simulink model "PDPWM_Three_Phase_Three_Level_Clamped_Inverter"  (R2022a)
settings: Solver=FixedStepAuto  StartTime=0.0  StopTime=0.3  FixedStep=1e-5  RelTol=1e-3
libraries: spsIGBTDiodeLib x12, spsDiodeLib x6, simulink x6, spsSeriesRLCBranchLib x5, spsGroundLib x2, spsDCVoltageSourceLib x1, spsThreePhaseVIMeasurementLib x1, spspowerguiLib x1
settings Model: Creator=nikos  LastModifiedBy=nikos

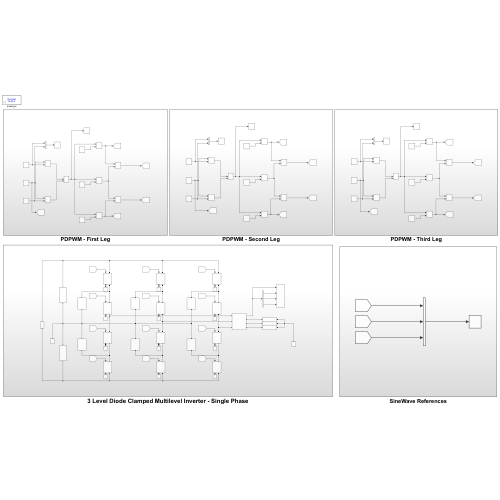
[thumbnail: Simulink's stored preview of the top-level diagram]
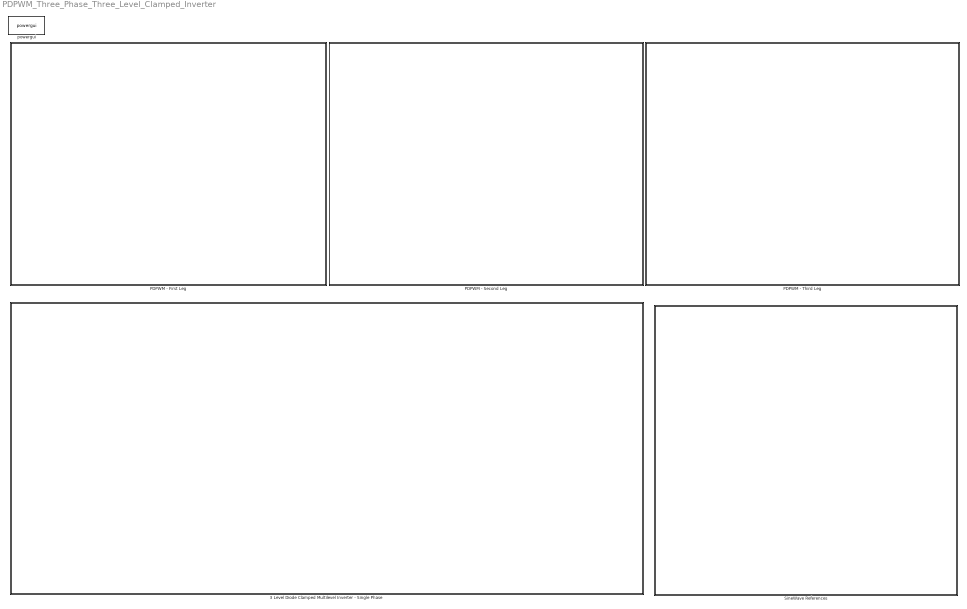
== system PDPWM_Three_Phase_Three_Level_Clamped_Inverter ==
  3 Level Diode Clamped Multilevel Inverter - Single Phase : Subsystem
  PDPWM - First Leg : Subsystem
  PDPWM - Second Leg : Subsystem
  PDPWM - Third Leg : Subsystem
  SineWave References : Subsystem
  powergui : spspowerguiLib/powergui  Priority=1  SimulationMode=Discrete  SampleTime=1e-5  frequency=60  Iterations=50  frequencyindice=0  Pbase=100e6  ErrMax=1e-4  UnitsV=kV  UnitsW=MW  buscounter=0  FunctionMessages=off  echomessages=off  EnableUseOfTLC=off  CurrentSourceSwitches=off  DisableSnubberDevices=off  DisableRonSwitches=off  DisableVfSwitches=off  DisplayEquations=off  AutomaticDiscreteSolvers=off  SolverType=Tustin/Backward Euler (TBE)  Interpol=off  ExternalGateDelay=off  methode=off  Ts=100  x0status=blocks  SPID=on  SwTol=0  HookPort=off  NonlinearTolerance=1e-4  nMaxIteration=100  ContinueOnMaxIteration=off  RestoreLinks=warning  ResistiveCurrentMeasurement=off  Frange=[0:2:500]  Ylog=off  Xlog=on  ShowGrid=off  save=off  variable=ZData  structure=0  ZoomFFT=off  StartTime=0.0  cycles=1  DisplayStyle=1  fundamental=60  FreqAxis=off  MaxFrequency=1000  frequencyindicesteady=1  RmsSteady=1  display=off

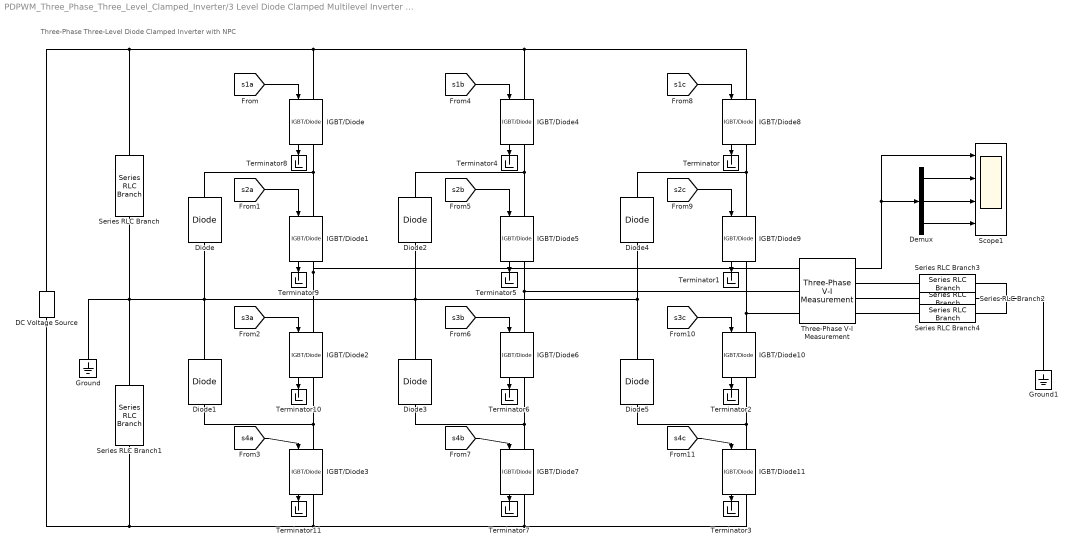
== system PDPWM_Three_Phase_Three_Level_Clamped_Inverter/3 Level Diode Clamped Multilevel Inverter - Single Phase ==
  note: Three-Phase Three-Level Diode Clamped Inverter with NPC
  DC Voltage Source : spsDCVoltageSourceLib/DC Voltage Source  Amplitude=100  Measurements=None
  Demux : Demux  Outputs=3
  Diode{,1..5} (6 alike) : spsDiodeLib/Diode  Ron=0.001  Lon=0  Vf=0.8  IC=0  UseSnubber=0  Rs=500  Cs=250e-9  Measurements=off
  Ground : spsGroundLib/Ground  LConnTagsString=a
  Ground1 : spsGroundLib/Ground  LConnTagsString=a
  IGBT/Diode{,1..11} (12 alike) : spsIGBTDiodeLib/IGBT//Diode  Ron=1e-3  Rs=1e5  Cs=inf  Measurements=on
  Scope1 : Scope  NumInputPorts=4
  Series RLC Branch : spsSeriesRLCBranchLib/Series RLC Branch  LConnTagsString=__new0  RConnTagsString=__new0  BranchType=RC  Resistance=0.01  Inductance=1e-3  SetiL0=off  InitialCurrent=0  Capacitance=4.7e-3  Setx0=off  InitialVoltage=0  Measurements=None
  Series RLC Branch1 : spsSeriesRLCBranchLib/Series RLC Branch  LConnTagsString=__new0  RConnTagsString=__new0  BranchType=RC  Resistance=0.01  Inductance=1e-3  SetiL0=off  InitialCurrent=0  Capacitance=4.7e-3  Setx0=off  InitialVoltage=0  Measurements=None
  Series RLC Branch2 : spsSeriesRLCBranchLib/Series RLC Branch  LConnTagsString=__new0  RConnTagsString=__new0  BranchType=R  Resistance=100  Inductance=1e-3  SetiL0=off  InitialCurrent=0  Capacitance=1e-6  Setx0=off  InitialVoltage=0  Measurements=None
  Series RLC Branch3 : spsSeriesRLCBranchLib/Series RLC Branch  LConnTagsString=__new0  RConnTagsString=__new0  BranchType=R  Resistance=100  Inductance=1e-3  SetiL0=off  InitialCurrent=0  Capacitance=1e-6  Setx0=off  InitialVoltage=0  Measurements=None
  Series RLC Branch4 : spsSeriesRLCBranchLib/Series RLC Branch  LConnTagsString=__new0  RConnTagsString=__new0  BranchType=R  Resistance=100  Inductance=1e-3  SetiL0=off  InitialCurrent=0  Capacitance=1e-6  Setx0=off  InitialVoltage=0  Measurements=None
  Terminator{,1..11} (12 alike) : Terminator
  Three-Phase V-I Measurement : spsThreePhaseVIMeasurementLib/Three-Phase V-I Measurement  VoltageMeasurement=phase-to-ground  SetLabelV=off  LabelV=Vabc  Vpu=off  VpuLL=off  CurrentMeasurement=no  SetLabelI=off  LabelI=Iabc  Ipu=off  Pbase=100e6  Vbase=500e3  OutputType=Complex  PhasorSimulation=off  PSBequivalent=0
  wires:
  [s4b] -> IGBT/Diode7/1
  [s2c] -> IGBT/Diode9/1
  Three-Phase V-I Measurement/1 -> Demux/1, Scope1/1
  Demux/3 -> Scope1/4
  [s3a] -> IGBT/Diode2/1
  [s3b] -> IGBT/Diode6/1
  [s2b] -> IGBT/Diode5/1
  [s1b] -> IGBT/Diode4/1
  [s4c] -> IGBT/Diode11/1
  [s2a] -> IGBT/Diode1/1
  [s1c] -> IGBT/Diode8/1
  [s1a] -> IGBT/Diode/1
  [s4a] -> IGBT/Diode3/1
  [s3c] -> IGBT/Diode10/1
  Demux/1 -> Scope1/2
  Demux/2 -> Scope1/3
  IGBT/Diode8/1 -> Terminator/1
  IGBT/Diode9/1 -> Terminator1/1
  IGBT/Diode10/1 -> Terminator2/1
  IGBT/Diode4/1 -> Terminator4/1
  IGBT/Diode5/1 -> Terminator5/1
  IGBT/Diode6/1 -> Terminator6/1
  IGBT/Diode7/1 -> Terminator7/1
  IGBT/Diode/1 -> Terminator8/1
  IGBT/Diode1/1 -> Terminator9/1
  IGBT/Diode2/1 -> Terminator10/1
  IGBT/Diode3/1 -> Terminator11/1
  IGBT/Diode11/1 -> Terminator3/1
  connections:
  IGBT/Diode7/LConn1 -- IGBT/Diode6/RConn1 -- Diode3/LConn1
  IGBT/Diode/RConn1 -- Diode/RConn1 -- IGBT/Diode1/LConn1
  Series RLC Branch1/RConn1 -- DC Voltage Source/LConn1 -- IGBT/Diode3/RConn1 -- IGBT/Diode7/RConn1 -- IGBT/Diode11/RConn1
  IGBT/Diode9/RConn1 -- Three-Phase V-I Measurement/LConn3 -- IGBT/Diode10/LConn1
  IGBT/Diode2/RConn1 -- Diode1/LConn1 -- IGBT/Diode3/LConn1
  IGBT/Diode5/LConn1 -- IGBT/Diode4/RConn1 -- Diode2/RConn1
  Series RLC Branch/RConn1 -- Ground/LConn1 -- Diode4/LConn1 -- Diode5/RConn1 -- Diode2/LConn1 -- Diode3/RConn1 -- Diode/LConn1 -- Diode1/RConn1 -- Series RLC Branch1/LConn1
  IGBT/Diode1/RConn1 -- IGBT/Diode2/LConn1 -- Three-Phase V-I Measurement/LConn1
  Series RLC Branch/LConn1 -- DC Voltage Source/RConn1 -- IGBT/Diode/LConn1 -- IGBT/Diode4/LConn1 -- IGBT/Diode8/LConn1
  IGBT/Diode5/RConn1 -- Three-Phase V-I Measurement/LConn2 -- IGBT/Diode6/LConn1
  IGBT/Diode10/RConn1 -- IGBT/Diode11/LConn1 -- Diode5/LConn1
  IGBT/Diode8/RConn1 -- IGBT/Diode9/LConn1 -- Diode4/RConn1
  Ground1/LConn1 -- Series RLC Branch4/LConn1 -- Series RLC Branch3/LConn1 -- Series RLC Branch2/LConn1
  Three-Phase V-I Measurement/RConn1 -- Series RLC Branch3/RConn1
  Three-Phase V-I Measurement/RConn3 -- Series RLC Branch4/RConn1
  Three-Phase V-I Measurement/RConn2 -- Series RLC Branch2/RConn1

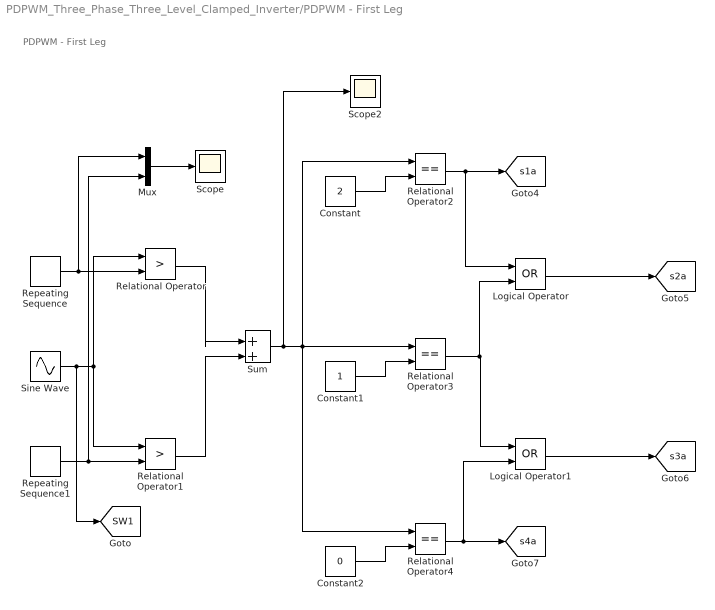
== system PDPWM_Three_Phase_Three_Level_Clamped_Inverter/PDPWM - First Leg ==
  note: PDPWM - First Leg
  Constant : Constant  Value=2
  Constant1 : Constant
  Constant2 : Constant  Value=0
  Logical Operator : Logic  Operator=OR  AllPortsSameDT=off  OutDataTypeStr=boolean
  Logical Operator1 : Logic  Operator=OR  AllPortsSameDT=off  OutDataTypeStr=boolean
  Mux : Mux  Inputs=2
  Relational Operator : RelationalOperator  Operator=>  OutDataTypeStr=boolean  RndMeth=Simplest  InputSameDT=off
  Relational Operator1 : RelationalOperator  Operator=>  OutDataTypeStr=boolean  RndMeth=Simplest  InputSameDT=off
  Relational Operator2 : RelationalOperator  Operator===  OutDataTypeStr=boolean  RndMeth=Simplest  InputSameDT=off
  Relational Operator3 : RelationalOperator  Operator===  OutDataTypeStr=boolean  RndMeth=Simplest  InputSameDT=off
  Relational Operator4 : RelationalOperator  Operator===  OutDataTypeStr=boolean  RndMeth=Simplest  InputSameDT=off
  Repeating Sequence : simulink/Sources/Repeating Sequence  rep_seq_t=[0 1 2]*[1/1000]  rep_seq_y=[0 1 0]
  Repeating Sequence1 : simulink/Sources/Repeating Sequence  rep_seq_t=[0 1 2]*[1/1000]  rep_seq_y=[-1 0 -1]
  Scope : Scope
  Scope2 : Scope
  Sine Wave : Sin  Frequency=2*pi*50  SampleTime=0
  Sum : Sum  Inputs=|++
  tag scope: SW1=global, s1a=global, s2a=global, s3a=global, s4a=global
  wires:
  Relational Operator3/1 -> Logical Operator/2, Logical Operator1/1
  Constant/1 -> Relational Operator2/2
  Repeating Sequence/1 -> Mux/1, Relational Operator/2
  Repeating Sequence1/1 -> Relational Operator1/2, Mux/2
  Relational Operator4/1 -> [s4a], Logical Operator1/2
  Relational Operator/1 -> Sum/1
  Relational Operator1/1 -> Sum/2
  Sine Wave/1 -> [SW1], Relational Operator1/1, Relational Operator/1
  Relational Operator2/1 -> [s1a], Logical Operator/1
  Mux/1 -> Scope/1
  Sum/1 -> Scope2/1, Relational Operator4/1, Relational Operator2/1, Relational Operator3/1
  Logical Operator/1 -> [s2a]
  Constant2/1 -> Relational Operator4/2
  Constant1/1 -> Relational Operator3/2
  Logical Operator1/1 -> [s3a]

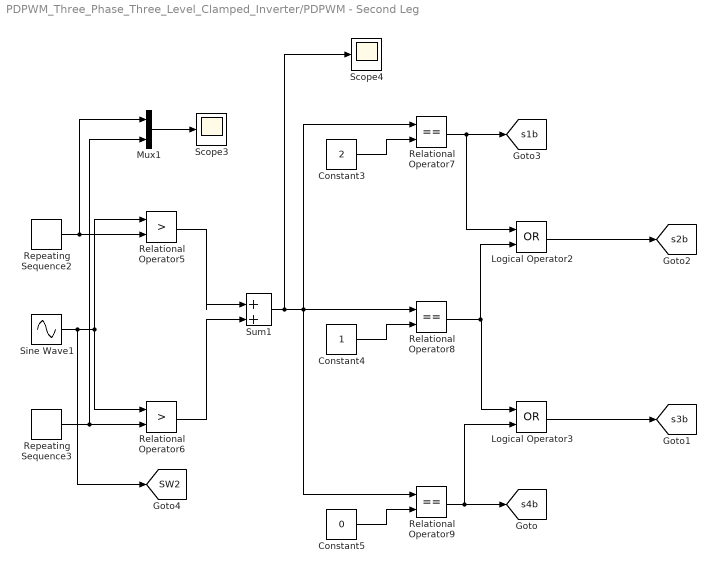
== system PDPWM_Three_Phase_Three_Level_Clamped_Inverter/PDPWM - Second Leg ==
  Constant3 : Constant  Value=2
  Constant4 : Constant
  Constant5 : Constant  Value=0
  Logical Operator2 : Logic  Operator=OR  AllPortsSameDT=off  OutDataTypeStr=boolean
  Logical Operator3 : Logic  Operator=OR  AllPortsSameDT=off  OutDataTypeStr=boolean
  Mux1 : Mux  Inputs=2
  Relational Operator5 : RelationalOperator  Operator=>  OutDataTypeStr=boolean  RndMeth=Simplest  InputSameDT=off
  Relational Operator6 : RelationalOperator  Operator=>  OutDataTypeStr=boolean  RndMeth=Simplest  InputSameDT=off
  Relational Operator7 : RelationalOperator  Operator===  OutDataTypeStr=boolean  RndMeth=Simplest  InputSameDT=off
  Relational Operator8 : RelationalOperator  Operator===  OutDataTypeStr=boolean  RndMeth=Simplest  InputSameDT=off
  Relational Operator9 : RelationalOperator  Operator===  OutDataTypeStr=boolean  RndMeth=Simplest  InputSameDT=off
  Repeating Sequence2 : simulink/Sources/Repeating Sequence  rep_seq_t=[0 1 2]*[1/1000]  rep_seq_y=[0 1 0]
  Repeating Sequence3 : simulink/Sources/Repeating Sequence  rep_seq_t=[0 1 2]*[1/1000]  rep_seq_y=[-1 0 -1]
  Scope3 : Scope
  Scope4 : Scope
  Sine Wave1 : Sin  Frequency=2*pi*50  Phase=4*pi/3  SampleTime=0
  Sum1 : Sum  Inputs=|++
  tag scope: SW2=global, s1b=global, s2b=global, s3b=global, s4b=global
  wires:
  Sum1/1 -> Relational Operator8/1, Relational Operator7/1, Relational Operator9/1, Scope4/1
  Relational Operator6/1 -> Sum1/2
  Relational Operator7/1 -> [s1b], Logical Operator2/1
  Logical Operator3/1 -> [s3b]
  Relational Operator5/1 -> Sum1/1
  Sine Wave1/1 -> [SW2], Relational Operator5/1, Relational Operator6/1
  Logical Operator2/1 -> [s2b]
  Relational Operator9/1 -> [s4b], Logical Operator3/2
  Relational Operator8/1 -> Logical Operator3/1, Logical Operator2/2
  Repeating Sequence3/1 -> Mux1/2, Relational Operator6/2
  Mux1/1 -> Scope3/1
  Constant3/1 -> Relational Operator7/2
  Constant4/1 -> Relational Operator8/2
  Constant5/1 -> Relational Operator9/2
  Repeating Sequence2/1 -> Relational Operator5/2, Mux1/1

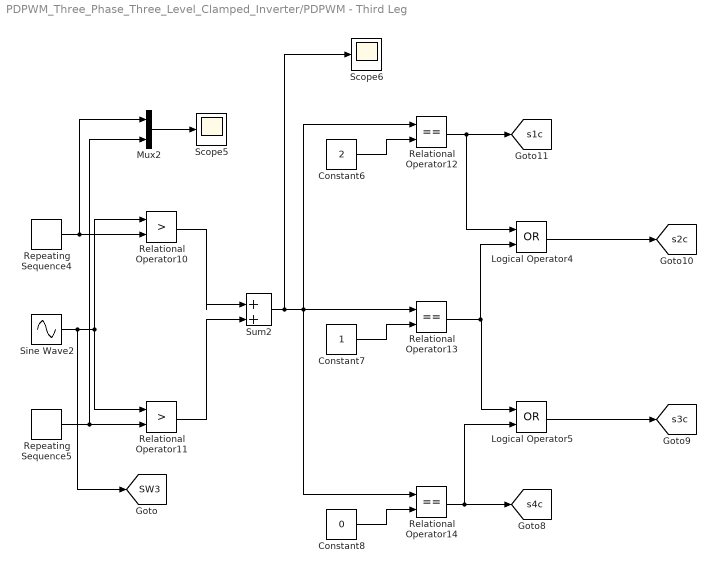
== system PDPWM_Three_Phase_Three_Level_Clamped_Inverter/PDPWM - Third Leg ==
  Constant6 : Constant  Value=2
  Constant7 : Constant
  Constant8 : Constant  Value=0
  Logical Operator4 : Logic  Operator=OR  AllPortsSameDT=off  OutDataTypeStr=boolean
  Logical Operator5 : Logic  Operator=OR  AllPortsSameDT=off  OutDataTypeStr=boolean
  Mux2 : Mux  Inputs=2
  Relational Operator10 : RelationalOperator  Operator=>  OutDataTypeStr=boolean  RndMeth=Simplest  InputSameDT=off
  Relational Operator11 : RelationalOperator  Operator=>  OutDataTypeStr=boolean  RndMeth=Simplest  InputSameDT=off
  Relational Operator12 : RelationalOperator  Operator===  OutDataTypeStr=boolean  RndMeth=Simplest  InputSameDT=off
  Relational Operator13 : RelationalOperator  Operator===  OutDataTypeStr=boolean  RndMeth=Simplest  InputSameDT=off
  Relational Operator14 : RelationalOperator  Operator===  OutDataTypeStr=boolean  RndMeth=Simplest  InputSameDT=off
  Repeating Sequence4 : simulink/Sources/Repeating Sequence  rep_seq_t=[0 1 2]*[1/1000]  rep_seq_y=[0 1 0]
  Repeating Sequence5 : simulink/Sources/Repeating Sequence  rep_seq_t=[0 1 2]*[1/1000]  rep_seq_y=[-1 0 -1]
  Scope5 : Scope
  Scope6 : Scope
  Sine Wave2 : Sin  Frequency=2*pi*50  Phase=2*pi/3  SampleTime=0
  Sum2 : Sum  Inputs=|++
  tag scope: SW3=global, s1c=global, s2c=global, s3c=global, s4c=global
  wires:
  Repeating Sequence5/1 -> Relational Operator11/2, Mux2/2
  Sine Wave2/1 -> [SW3], Relational Operator11/1, Relational Operator10/1
  Repeating Sequence4/1 -> Mux2/1, Relational Operator10/2
  Constant8/1 -> Relational Operator14/2
  Logical Operator5/1 -> [s3c]
  Relational Operator11/1 -> Sum2/2
  Relational Operator12/1 -> [s1c], Logical Operator4/1
  Logical Operator4/1 -> [s2c]
  Sum2/1 -> Scope6/1, Relational Operator14/1, Relational Operator12/1, Relational Operator13/1
  Relational Operator14/1 -> [s4c], Logical Operator5/2
  Relational Operator10/1 -> Sum2/1
  Constant7/1 -> Relational Operator13/2
  Constant6/1 -> Relational Operator12/2
  Mux2/1 -> Scope5/1
  Relational Operator13/1 -> Logical Operator4/2, Logical Operator5/1

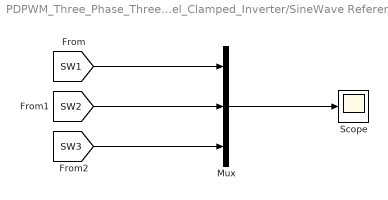
== system PDPWM_Three_Phase_Three_Level_Clamped_Inverter/SineWave References ==
  Mux : Mux  Inputs=3
  Scope : Scope
  wires:
  [SW1] -> Mux/1
  [SW2] -> Mux/2
  Mux/1 -> Scope/1
  [SW3] -> Mux/3
